simulink model "SimulacaoSala"  (R2017b)
settings: Solver=VariableStepAuto  StartTime=0.0  StopTime=14000  RelTol=1e-3
values from neighbouring files (symbols this model uses):
  A = [1.00413840626  -0.0299276874599; 0.059623507209  0.940484886129]    [SimulacaoSalaDados.mat]
  B = [-0.000104228584218 0.00212022584315]    [SimulacaoSalaDados.mat]
  C = [49.9995779895 1.24069988178]    [SimulacaoSalaDados.mat]
  D = 0    [SimulacaoSalaDados.mat]
libraries: mpclib x1
settings Model: Creator=heyderaraujo  LastModifiedBy=heyderaraujo

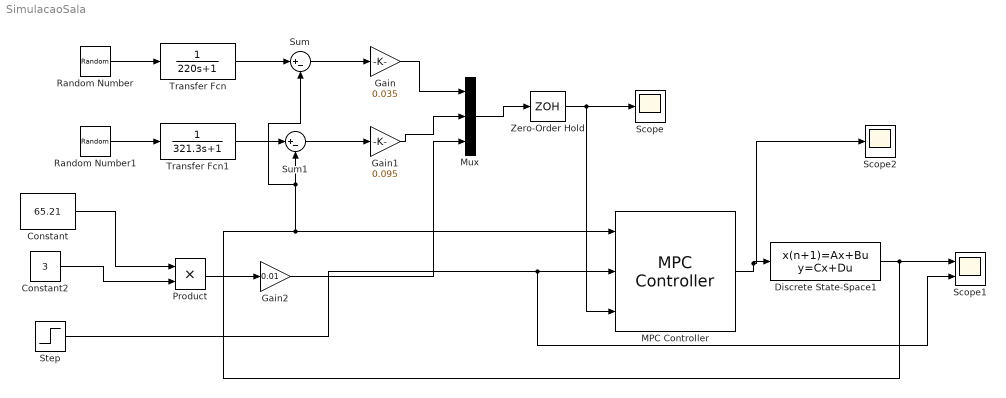
== system SimulacaoSala ==
  Constant : Constant  Value=65.21
  Constant2 : Constant  Value=3
  Discrete State-Space1 : DiscreteStateSpace  A=A  B=B  C=C  D=D  SampleTime=-1
  Gain : Gain  Gain=0.035
  Gain1 : Gain  Gain=0.095
  Gain2 : Gain  Gain=0.01
  MPC Controller : mpclib/MPC Controller  SCDEnableBlockLinearizationSpecification=on  mpcobj=mpc1  is_multiple=0  enable_value=0  return_u0=off  ref_from_ws=off  ref_signal_name=[]  ref_preview=off  md_from_ws=off  md_signal_name=[]  md_preview=off  from_project=off  project_file=MPCtask.mat  md_inport=on  mv_inport=off  cost_outport=off  return_sequence=off  return_qpstatus=off  return_state=off  state_inport=off  lims_inport=off  cc_inport=off  ywt_inport=off  is_designfromscratch=0  uwt_inport=off  duwt_inport=off  rhoeps_inport=off  uref_inport=off  n_ts=1  n_p=30  n_mv=1  n_md=1  n_ud=0  n_mo=1  n_uo=0  BlockDataType=double  SampleTimeInherited=off  switch_inport=off
  Mux : Mux  Inputs=3
  Product : Product
  Random Number : RandomNumber  Mean=30  Seed=1  SampleTime=0.1
  Random Number1 : RandomNumber  Mean=24  Seed=1  SampleTime=0.1
  Scope : Scope
  Scope1 : Scope  NumInputPorts=2
  Scope2 : Scope
  Step : Step  Time=320  Before=30  After=21.5  SampleTime=0
  Sum : Sum  Inputs=|+-
  Sum1 : Sum  Inputs=|+-
  Transfer Fcn : TransferFcn  Denominator=[220 1]
  Transfer Fcn1 : TransferFcn  Denominator=[321.3 1]
  Zero-Order Hold : ZeroOrderHold  SampleTime=-1
  wires:
  Random Number/1 -> Transfer Fcn/1
  Random Number1/1 -> Transfer Fcn1/1
  Transfer Fcn1/1 -> Sum1/1
  Transfer Fcn/1 -> Sum/1
  Discrete State-Space1/1 -> Scope1/1, Sum/2, Sum1/2, MPC Controller/1
  Sum/1 -> Gain/1
  Sum1/1 -> Gain1/1
  Gain/1 -> Mux/1
  Gain1/1 -> Mux/2
  Constant/1 -> Product/1
  Constant2/1 -> Product/2
  Product/1 -> Gain2/1
  Step/1 -> Scope1/2, MPC Controller/2
  Zero-Order Hold/1 -> MPC Controller/3, Scope/1
  MPC Controller/1 -> Scope2/1, Discrete State-Space1/1
  Gain2/1 -> Mux/3
  Mux/1 -> Zero-Order Hold/1
